simulink model "abslut50_fixpt20_32"  (R2021b)
settings: Solver=VariableStepAuto  StartTime=0.0  StopTime=99  RelTol=1e-3
undefined symbols (not defined in the file or in its folder): figd2104, xcu250
libraries: hdlBasic x5226, vmcUtilities x1
(part 1 of 17)
settings Model: Creator=shu_abe  LastModifiedBy=shu_abe

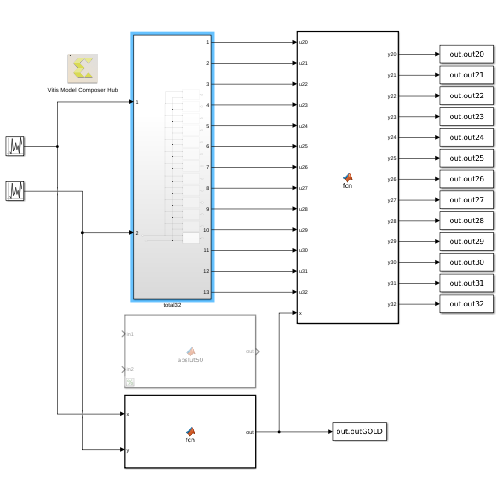
[thumbnail: Simulink's stored preview of the top-level diagram]
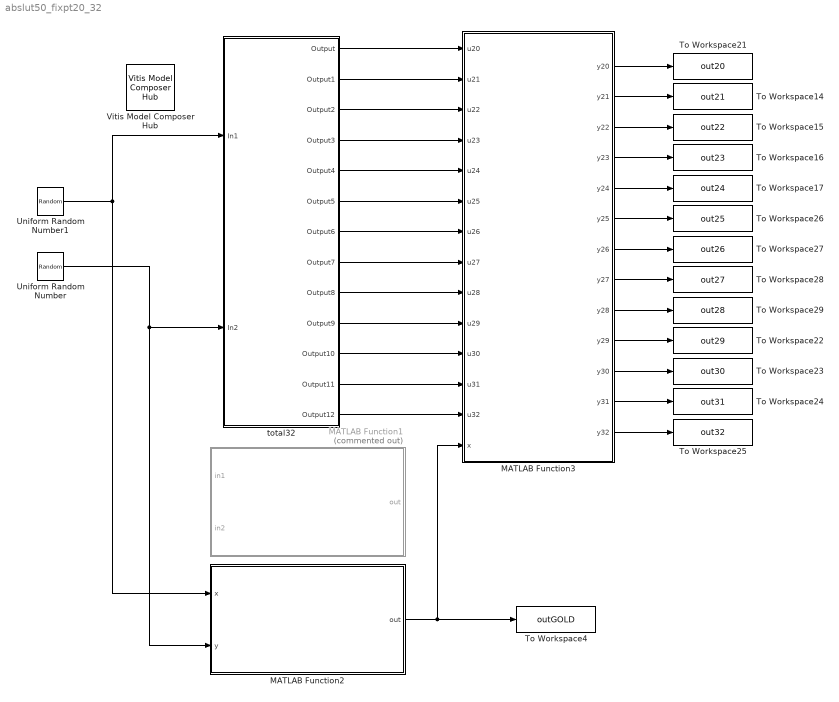
== system abslut50_fixpt20_32 ==
  MATLAB Function1 : MATLAB Function  Commented=on  TreatAsAtomicUnit=on
  MATLAB Function2 : MATLAB Function  TreatAsAtomicUnit=on
  MATLAB Function3 : MATLAB Function  TreatAsAtomicUnit=on
  To Workspace14 : ToWorkspace  VariableName=out21  SaveFormat=Structure With Time  SampleTime=-1
  To Workspace15 : ToWorkspace  VariableName=out22  SaveFormat=Structure With Time  SampleTime=-1
  To Workspace16 : ToWorkspace  VariableName=out23  SaveFormat=Structure With Time  SampleTime=-1
  To Workspace17 : ToWorkspace  VariableName=out24  SaveFormat=Structure With Time  SampleTime=-1
  To Workspace21 : ToWorkspace  VariableName=out20  SaveFormat=Structure With Time  SampleTime=-1
  To Workspace22 : ToWorkspace  VariableName=out29  SaveFormat=Structure With Time  SampleTime=-1
  To Workspace23 : ToWorkspace  VariableName=out30  SaveFormat=Structure With Time  SampleTime=-1
  To Workspace24 : ToWorkspace  VariableName=out31  SaveFormat=Structure With Time  SampleTime=-1
  To Workspace25 : ToWorkspace  VariableName=out32  SaveFormat=Structure With Time  SampleTime=-1
  To Workspace26 : ToWorkspace  VariableName=out25  SaveFormat=Structure With Time  SampleTime=-1
  To Workspace27 : ToWorkspace  VariableName=out26  SaveFormat=Structure With Time  SampleTime=-1
  To Workspace28 : ToWorkspace  VariableName=out27  SaveFormat=Structure With Time  SampleTime=-1
  To Workspace29 : ToWorkspace  VariableName=out28  SaveFormat=Structure With Time  SampleTime=-1
  To Workspace4 : ToWorkspace  VariableName=outGOLD  SaveFormat=Structure With Time  SampleTime=1
  Uniform Random Number : UniformRandomNumber  Minimum=-0.9  Maximum=0.9  SampleTime=1
  Uniform Random Number1 : UniformRandomNumber  Minimum=-0.9  Maximum=0.9  Seed=1  SampleTime=1
  Vitis Model Composer Hub : vmcUtilities/Vitis Model Composer Hub  Tag=genX  CodeGeneration=off  SubsystemName=<enter or select subsystem name>  TargetDirectory=./code  ExportType=HLS C++ code  IpVendor=xilinx.com  IpLibrary=hls  IpVersion=1.0  IpHWLanguage=Verilog  AieCompilerOptions={}  CreateTestbench=off  TestbenchStackSize=10  RunAieSim=off  AieSimTimeout=50000  RunAieSimProfiling=off  LaunchVitisAnalyzer=off  PlotOutput=off  RunX86Sim=off  X86SimTimeout=10  GenHwImage=off  PlatformType=Not Specified  HwSystemType=Baremetal  HwValidationTarget=hw  ProjDevice=Alveo U250 Data Center Accelerator Card (xcu250-figd2104-2L-e)  ProjDevicePart=xcu250-figd2104-2L-e  SamplePeriod=-1  ClockFrequency=200  DataPathParallelism=1  xilinxfamily=virtexuplus  part=xcu250  speed=-2L-e  package=figd2104  directory=./abslut50_fixpt32  testbench=off  incr_netlist=off  synthesis_tool=Vivado  clock_wrapper=Clock Enables  dbl_ovrd=According to Block Masks  dcm_input_clock_period=10  sysclk_period=50  simulink_period=1  eval_field=0
  total32 : Subsystem
  wires:
  MATLAB Function2/1(out) -> MATLAB Function3/14(x), To Workspace4/1
  Uniform Random Number1/1 -> MATLAB Function2/1(x), total32/1(In1)
  Uniform Random Number/1 -> MATLAB Function2/2(y), total32/2(In2)
  MATLAB Function3/11(y30) -> To Workspace23/1
  MATLAB Function3/2(y21) -> To Workspace14/1
  MATLAB Function3/13(y32) -> To Workspace25/1
  MATLAB Function3/12(y31) -> To Workspace24/1
  MATLAB Function3/8(y27) -> To Workspace28/1
  MATLAB Function3/9(y28) -> To Workspace29/1
  MATLAB Function3/10(y29) -> To Workspace22/1
  MATLAB Function3/5(y24) -> To Workspace17/1
  MATLAB Function3/6(y25) -> To Workspace26/1
  MATLAB Function3/7(y26) -> To Workspace27/1
  MATLAB Function3/3(y22) -> To Workspace15/1
  MATLAB Function3/4(y23) -> To Workspace16/1
  MATLAB Function3/1(y20) -> To Workspace21/1
  total32/1(Output) -> MATLAB Function3/1(u20)
  total32/2(Output1) -> MATLAB Function3/2(u21)
  total32/3(Output2) -> MATLAB Function3/3(u22)
  total32/4(Output3) -> MATLAB Function3/4(u23)
  total32/5(Output4) -> MATLAB Function3/5(u24)
  total32/6(Output5) -> MATLAB Function3/6(u25)
  total32/7(Output6) -> MATLAB Function3/7(u26)
  total32/8(Output7) -> MATLAB Function3/8(u27)
  total32/9(Output8) -> MATLAB Function3/9(u28)
  total32/10(Output9) -> MATLAB Function3/10(u29)
  total32/11(Output10) -> MATLAB Function3/11(u30)
  total32/12(Output11) -> MATLAB Function3/12(u31)
  total32/13(Output12) -> MATLAB Function3/13(u32)

== system abslut50_fixpt20_32/total32 ==
  In1 : Inport
  In2 : Inport  Port=2
  Subsystem20bit : Subsystem
  Subsystem21bit : Subsystem
  Subsystem22bit : Subsystem
  Subsystem23bit : Subsystem
  Subsystem24bit : Subsystem
  Subsystem25bit : Subsystem
  Subsystem26bit : Subsystem
  Subsystem27bit : Subsystem
  Subsystem28bit : Subsystem
  Subsystem29bit : Subsystem
  Subsystem30bit : Subsystem
  Subsystem31bit : Subsystem
  Subsystem32bit : Subsystem
  Output : Outport
  Output1 : Outport  Port=2
  Output2 : Outport  Port=3
  Output3 : Outport  Port=4
  Output4 : Outport  Port=5
  Output5 : Outport  Port=6
  Output6 : Outport  Port=7
  Output7 : Outport  Port=8
  Output8 : Outport  Port=9
  Output9 : Outport  Port=10
  Output10 : Outport  Port=11
  Output11 : Outport  Port=12
  Output12 : Outport  Port=13
  wires:
  Subsystem29bit/1(Output) -> Output9/1
  Subsystem25bit/1(Output) -> Output5/1
  Subsystem32bit/1(Output) -> Output12/1
  Subsystem23bit/1(Output) -> Output3/1
  Subsystem20bit/1(Output) -> Output/1
  Subsystem22bit/1(Output) -> Output2/1
  Subsystem21bit/1(Output) -> Output1/1
  Subsystem26bit/1(Output) -> Output6/1
  Subsystem24bit/1(Output) -> Output4/1
  In2/1 -> Subsystem29bit/2(In4), Subsystem28bit/2(In4), Subsystem27bit/2(In4), Subsystem26bit/2(In4), Subsystem25bit/2(In4), Subsystem23bit/2(In4), Subsystem20bit/2(In4), Subsystem21bit/2(In4), Subsystem22bit/2(In4), Subsystem24bit/2(In4), Subsystem30bit/2(In4), Subsystem31bit/2(In4), Subsystem32bit/2(In4)
  Subsystem30bit/1(Output) -> Output10/1
  Subsystem28bit/1(Output) -> Output8/1
  Subsystem27bit/1(Output) -> Output7/1
  Subsystem31bit/1(Output) -> Output11/1
  In1/1 -> Subsystem30bit/1(In3), Subsystem28bit/1(In3), Subsystem26bit/1(In3), Subsystem25bit/1(In3), Subsystem24bit/1(In3), Subsystem23bit/1(In3), Subsystem20bit/1(In3), Subsystem21bit/1(In3), Subsystem22bit/1(In3), Subsystem27bit/1(In3), Subsystem29bit/1(In3), Subsystem31bit/1(In3), Subsystem32bit/1(In3)
